simulink model "increase_pid"  (R2019a)
settings: Solver=VariableStepAuto  StartTime=0.0  StopTime=50  RelTol=1e-3
settings Model: Creator=intel  LastModifiedBy=intel

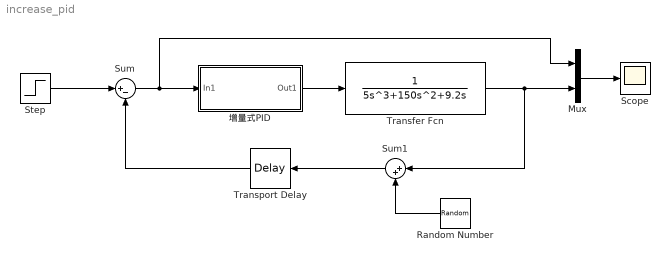
== system increase_pid ==
  Mux : Mux  Inputs=2
  Random Number : RandomNumber  SampleTime=0.1
  Scope : Scope
  Step : Step  After=40  SampleTime=0
  Sum : Sum  Inputs=|+-
  Sum1 : Sum  Inputs=|++
  Transfer Fcn : TransferFcn  Denominator=[5 150 9.2 0]
  Transport Delay : TransportDelay  DelayTime=0.02
  增量式PID : Subsystem
  wires:
  Step/1 -> Sum/1
  Sum/1 -> Mux/1, 增量式PID/1(In1)
  增量式PID/1(Out1) -> Transfer Fcn/1
  Transfer Fcn/1 -> Sum1/1, Mux/2
  Random Number/1 -> Sum1/2
  Mux/1 -> Scope/1
  Sum1/1 -> Transport Delay/1
  Transport Delay/1 -> Sum/2

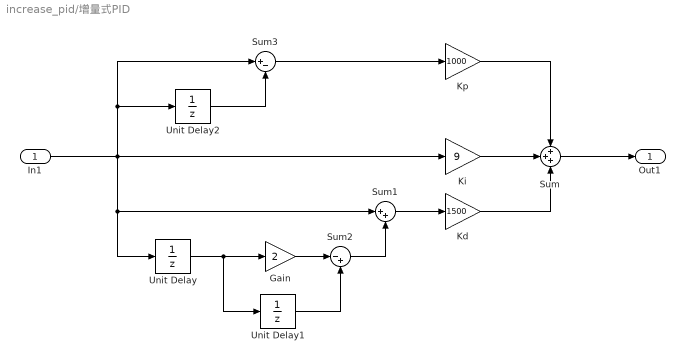
== system increase_pid/增量式PID ==
  In1 : Inport
  Gain : Gain  Gain=2
  Kd : Gain  Gain=1500
  Ki : Gain  Gain=9
  Kp : Gain  Gain=1000
  Sum : Sum  Inputs=+++
  Sum1 : Sum  Inputs=|++
  Sum2 : Sum  Inputs=|-+
  Sum3 : Sum  Inputs=|+-
  Unit Delay : UnitDelay  SampleTime=0.02  HasFrameUpgradeWarning=on
  Unit Delay1 : UnitDelay  SampleTime=0.02  HasFrameUpgradeWarning=on
  Unit Delay2 : UnitDelay  SampleTime=0.02  HasFrameUpgradeWarning=on
  Out1 : Outport
  wires:
  Gain/1 -> Sum2/1
  In1/1 -> Sum1/1, Unit Delay/1, Ki/1, Unit Delay2/1, Sum3/1
  Sum3/1 -> Kp/1
  Sum1/1 -> Kd/1
  Unit Delay2/1 -> Sum3/2
  Sum2/1 -> Sum1/2
  Unit Delay/1 -> Unit Delay1/1, Gain/1
  Unit Delay1/1 -> Sum2/2
  Ki/1 -> Sum/2
  Kp/1 -> Sum/1
  Kd/1 -> Sum/3
  Sum/1 -> Out1/1
